simulink model "position"  (R2019b)
settings: Solver=VariableStepAuto  StartTime=0.0  StopTime=10.0  RelTol=1e-3
values from neighbouring files (symbols this model uses):
  b = 2.18e-6    (= 2.18e-06)    [OpenCalc.m]    (also in OpenLoop.m = 0.1; model.m = 0.00073)
  J = 22.519e-7    (= 2.2519e-06)    [OpenCalc.m]    (also in OpenLoop.m = 0.01; model.m = 2.25e-06)
  K = 42.9e-3    (= 0.0429)    [OpenCalc.m]    (also in OpenLoop.m = 0.01; model.m)
  L = 0.514e-3    (= 0.000514)    [OpenCalc.m]    (also in OpenLoop.m = 5; model.m)
  R = 2.68    [OpenCalc.m]    (also in OpenLoop.m = 1; model.m)
libraries: simulink x1
settings Model: Creator=chris  LastModifiedBy=chris

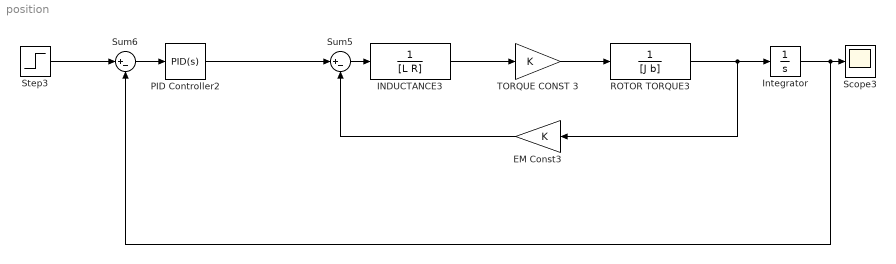
== system position ==
  EM Const3 : Gain  Gain=K
  INDUCTANCE3 : TransferFcn  Denominator=[L R]
  Integrator : Integrator
  PID Controller2 : simulink/Continuous/PID Controller  Controller=PID  Form=Parallel  TimeDomain=Continuous-time  SampleTime=-1  IntegratorMethod=Forward Euler  FilterMethod=Forward Euler  ControllerParametersSource=internal  P=1  I=0  D=0  UseFilter=on  N=100  TunerSelectOption=Transfer Function Based (PID Tuner App)  InitialConditionSource=internal  InitialConditionForIntegrator=0  InitialConditionForFilter=0  DifferentiatorICPrevScaledInput=0  ExternalReset=none  TrackingMode=off  Kt=1  LimitOutput=off  UpperSaturationLimit=inf  LowerSaturationLimit=-inf  LinearizeAsGain=on  AntiWindupMode=none  Kb=1  POutMin=[]  POutMax=[]  IOutMin=[]  IOutMax=[]  DOutMin=[]  DOutMax=[]  NOutMin=[]  NOutMax=[]  SumOutMin=[]  SumOutMax=[]  SaturationOutMin=[]  SaturationOutMax=[]  PParamMin=[]  PParamMax=[]  IParamMin=[]  IParamMax=[]  DParamMin=[]  DParamMax=[]  NParamMin=[]  NParamMax=[]  KbParamMin=[]  KbParamMax=[]  KtParamMin=[]  KtParamMax=[]  KbOutMin=[]  KbOutMax=[]  KtOutMin=[]  KtOutMax=[]  IntegratorOutMin=[]  IntegratorOutMax=[]  FilterOutMin=[]  FilterOutMax=[]  SumI1OutMin=[]  SumI1OutMax=[]  SumI2OutMin=[]  SumI2OutMax=[]  SumI3OutMin=[]  SumI3OutMax=[]  SumI4OutMin=[]  SumI4OutMax=[]  SumDOutMin=[]  SumDOutMax=[]  DifferentiatorOutMin=[]  DifferentiatorOutMax=[]  FilterDiffOutCoefMin=[]  FilterDiffOutCoefMax=[]  ReciprocalOutMin=[]  ReciprocalOutMax=[]  SumDenOutMin=[]  SumDenOutMax=[]  SumNumOutMin=[]  SumNumOutMax=[]  DivideOutMin=[]  DivideOutMax=[]  IntegratorContinuousStateAttributes=''  IntegratorStateMustResolveToSignalObject=off  IntegratorRTWStateStorageClass=Auto  FilterContinuousStateAttributes=''  FilterStateMustResolveToSignalObject=off  FilterRTWStateStorageClass=Auto  ParallelPVariant=InternalParameters  IdealPVariant=Disabled  IVariant=InternalParameters  DVariant=InternalParameters  IntegratorVariant=Continuous  SatVariant=Disabled  AWVariant=Passthrough  PCopyVariant=Disabled  TRVariant=Disabled  FdbkBlocksVariant=Forward  IdealPFdbkVariant=Disabled  SatFdbkVariant=Disabled  DerivativeFilterVariant=ContFilter  NVariant=InternalParameters  NCopyVariant=Disabled  FilterICVariant=InternalICsFilter  IntegratorICVariant=InternalICs  ExternalResetVariant=Disabled  TRSumVariant=Passthrough  SumFdbkVariant=Disabled  SumVariant=Sum_PID
  ROTOR TORQUE3 : TransferFcn  Denominator=[J b]
  Scope3 : Scope
  Step3 : Step  Time=0  SampleTime=0
  Sum5 : Sum  Inputs=|+-
  Sum6 : Sum  Inputs=|+-
  TORQUE CONST 3 : Gain  Gain=K
  wires:
  Integrator/1 -> Scope3/1, Sum6/2
  Sum6/1 -> PID Controller2/1
  Step3/1 -> Sum6/1
  ROTOR TORQUE3/1 -> EM Const3/1, Integrator/1
  Sum5/1 -> INDUCTANCE3/1
  TORQUE CONST 3/1 -> ROTOR TORQUE3/1
  INDUCTANCE3/1 -> TORQUE CONST 3/1
  EM Const3/1 -> Sum5/2
  PID Controller2/1 -> Sum5/1
